simulink model "model"  (R2014a)
(part 5 of 5)

  T_195060971_110000_Подстанция_«Игольская»/RConn1 -- L_195060971/LConn1
  T_195060971_110000_Подстанция_«Игольская»/RConn2 -- L_195060971/LConn2
  L_195060971/LConn3 -- T_195060971_110000_Подстанция_«Игольская»/RConn3 -- bus396/LConn1
  T_332123970__/RConn1 -- L_332123970/LConn1
  T_332123970__/RConn2 -- L_332123970/LConn2
  L_332123970/LConn3 -- T_332123970__/RConn3 -- bus397/LConn1
  T_332122569__/RConn1 -- L_332122569/LConn1
  T_332122569__/RConn2 -- L_332122569/LConn2
  L_332122569/LConn3 -- T_332122569__/RConn3 -- bus398/LConn1
  T_194874204_110000_Подстанция_«Крапивинская»/RConn1 -- L_194874204/LConn1
  T_194874204_110000_Подстанция_«Крапивинская»/RConn2 -- L_194874204/LConn2
  L_194874204/LConn3 -- T_194874204_110000_Подстанция_«Крапивинская»/RConn3 -- bus399/LConn1
  T_100718452__Ефремовская/RConn1 -- L_100718452/LConn1
  T_100718452__Ефремовская/RConn2 -- L_100718452/LConn2
  L_100718452/LConn3 -- T_100718452__Ефремовская/RConn3 -- bus400/LConn1
  T_94337786__Оловозаводская/RConn1 -- L_94337786/LConn1
  T_94337786__Оловозаводская/RConn2 -- L_94337786/LConn2
  L_94337786/LConn3 -- T_94337786__Оловозаводская/RConn3 -- bus401/LConn1
  T_201600394_110000_Подстанция_«Верх_Угрюм»/RConn1 -- L_201600394/LConn1
  T_201600394_110000_Подстанция_«Верх_Угрюм»/RConn2 -- L_201600394/LConn2
  L_201600394/LConn3 -- T_201600394_110000_Подстанция_«Верх_Угрюм»/RConn3 -- bus402/LConn1
  T_203056539__Тяговая_ПС_Суховская/RConn1 -- L_203056539/LConn1
  T_203056539__Тяговая_ПС_Суховская/RConn2 -- L_203056539/LConn2
  L_203056539/LConn3 -- T_203056539__Тяговая_ПС_Суховская/RConn3 -- bus403/LConn1
  T_298817867__/RConn1 -- L_298817867/LConn1
  T_298817867__/RConn2 -- L_298817867/LConn2
  L_298817867/LConn3 -- T_298817867__/RConn3 -- bus404/LConn1
  T_367574444__/RConn1 -- L_367574444/LConn1
  T_367574444__/RConn2 -- L_367574444/LConn2
  L_367574444/LConn3 -- T_367574444__/RConn3 -- bus405/LConn1
  T_283373486__/RConn1 -- L_283373486/LConn1
  T_283373486__/RConn2 -- L_283373486/LConn2
  L_283373486/LConn3 -- T_283373486__/RConn3 -- bus406/LConn1
  "T_110542603_220000_ПС_№152_\"Новокрасноярская\""/RConn1 -- L_110542603/LConn1
  "T_110542603_220000_ПС_№152_\"Новокрасноярская\""/RConn2 -- L_110542603/LConn2
  L_110542603/LConn3 -- "T_110542603_220000_ПС_№152_\"Новокрасноярская\""/RConn3 -- bus407/LConn1
  T_116607512__/RConn1 -- L_116607512/LConn1
  T_116607512__/RConn2 -- L_116607512/LConn2
  L_116607512/LConn3 -- T_116607512__/RConn3 -- bus408/LConn1
  T_394149419_220000_Подстанция_«Орловка»/RConn1 -- L_394149419/LConn1
  T_394149419_220000_Подстанция_«Орловка»/RConn2 -- L_394149419/LConn2
  L_394149419/LConn3 -- T_394149419_220000_Подстанция_«Орловка»/RConn3 -- bus409/LConn1
  T_166018985_500000_Подстанция_«Томская»/RConn1 -- L_166018985/LConn1
  T_166018985_500000_Подстанция_«Томская»/RConn2 -- L_166018985/LConn2
  L_166018985/LConn3 -- T_166018985_500000_Подстанция_«Томская»/RConn3 -- bus410/LConn1
  T_48050742_220000_ПС_ЦРП_220_кВ/RConn1 -- L_48050742/LConn1
  T_48050742_220000_ПС_ЦРП_220_кВ/RConn2 -- L_48050742/LConn2
  L_48050742/LConn3 -- T_48050742_220000_ПС_ЦРП_220_кВ/RConn3 -- bus411/LConn1
  T_220574879_220000_ОРУ___ГПП_3/RConn1 -- L_220574879/LConn1
  T_220574879_220000_ОРУ___ГПП_3/RConn2 -- L_220574879/LConn2
  L_220574879/LConn3 -- T_220574879_220000_ОРУ___ГПП_3/RConn3 -- bus412/LConn1
  T_60040500_220000_ОРУ___ГПП_5/RConn1 -- L_60040500/LConn1
  T_60040500_220000_ОРУ___ГПП_5/RConn2 -- L_60040500/LConn2
  L_60040500/LConn3 -- T_60040500_220000_ОРУ___ГПП_5/RConn3 -- bus413/LConn1
  T_60040415_220000_ОРУ___ГПП_1/RConn1 -- L_60040415/LConn1
  T_60040415_220000_ОРУ___ГПП_1/RConn2 -- L_60040415/LConn2
  L_60040415/LConn3 -- T_60040415_220000_ОРУ___ГПП_1/RConn3 -- bus414/LConn1
  "T_105828925_220000;110000;10000_ПС_\"Узловая\""/RConn1 -- L_105828925/LConn1
  "T_105828925_220000;110000;10000_ПС_\"Узловая\""/RConn2 -- L_105828925/LConn2
  L_105828925/LConn3 -- "T_105828925_220000;110000;10000_ПС_\"Узловая\""/RConn3 -- bus415/LConn1
  T_435735615_220000_ОРУ_220_кВ/RConn1 -- L_435735615/LConn1
  T_435735615_220000_ОРУ_220_кВ/RConn2 -- L_435735615/LConn2
  L_435735615/LConn3 -- T_435735615_220000_ОРУ_220_кВ/RConn3 -- bus416/LConn1
  T_221635306__Подстанция_«Сорская»/RConn1 -- L_221635306/LConn1
  T_221635306__Подстанция_«Сорская»/RConn2 -- L_221635306/LConn2
  L_221635306/LConn3 -- T_221635306__Подстанция_«Сорская»/RConn3 -- bus417/LConn1
  T_228972838__/RConn1 -- L_228972838/LConn1
  T_228972838__/RConn2 -- L_228972838/LConn2
  L_228972838/LConn3 -- T_228972838__/RConn3 -- bus418/LConn1
  T_113629981_220000;110000;35000;fixme_/RConn1 -- L_113629981/LConn1
  T_113629981_220000;110000;35000;fixme_/RConn2 -- L_113629981/LConn2
  L_113629981/LConn3 -- T_113629981_220000;110000;35000;fixme_/RConn3 -- bus419/LConn1
  T_228023756_220000_Подстанция_«Вертикос»/RConn1 -- L_228023756/LConn1
  T_228023756_220000_Подстанция_«Вертикос»/RConn2 -- L_228023756/LConn2
  L_228023756/LConn3 -- T_228023756_220000_Подстанция_«Вертикос»/RConn3 -- bus420/LConn1
  T_245816959__/RConn1 -- L_245816959/LConn1
  T_245816959__/RConn2 -- L_245816959/LConn2
  L_245816959/LConn3 -- T_245816959__/RConn3 -- bus421/LConn1
  T_60040328_220000_ОРУ___ГПП_4/RConn1 -- L_60040328/LConn1
  T_60040328_220000_ОРУ___ГПП_4/RConn2 -- L_60040328/LConn2
  L_60040328/LConn3 -- T_60040328_220000_ОРУ___ГПП_4/RConn3 -- bus422/LConn1
  T_116489400__/RConn1 -- L_116489400/LConn1
  T_116489400__/RConn2 -- L_116489400/LConn2
  L_116489400/LConn3 -- T_116489400__/RConn3 -- bus423/LConn1
  T_60040606_220000_ОРУ___ГПП_2/RConn1 -- L_60040606/LConn1
  T_60040606_220000_ОРУ___ГПП_2/RConn2 -- L_60040606/LConn2
  L_60040606/LConn3 -- T_60040606_220000_ОРУ___ГПП_2/RConn3 -- bus424/LConn1
  T_341189940__/RConn1 -- L_341189940/LConn1
  T_341189940__/RConn2 -- L_341189940/LConn2
  L_341189940/LConn3 -- T_341189940__/RConn3 -- bus425/LConn1
  T_166616387__ЭС_2_СХК/RConn1 -- L_166616387/LConn1
  T_166616387__ЭС_2_СХК/RConn2 -- L_166616387/LConn2
  L_166616387/LConn3 -- T_166616387__ЭС_2_СХК/RConn3 -- bus426/LConn1
  T_131753194_220000;110000;10000_Абакан_Районная/RConn1 -- L_131753194/LConn1
  T_131753194_220000;110000;10000_Абакан_Районная/RConn2 -- L_131753194/LConn2
  L_131753194/LConn3 -- T_131753194_220000;110000;10000_Абакан_Районная/RConn3 -- bus427/LConn1
  T_115163974_220000_Подстанция_«Минусинск_Опорная»/RConn1 -- L_115163974/LConn1
  T_115163974_220000_Подстанция_«Минусинск_Опорная»/RConn2 -- L_115163974/LConn2
  L_115163974/LConn3 -- T_115163974_220000_Подстанция_«Минусинск_Опорная»/RConn3 -- bus428/LConn1
  "T_60040448_220000_РПС_\"КРАМЗ\""/RConn1 -- L_60040448/LConn1
  "T_60040448_220000_РПС_\"КРАМЗ\""/RConn2 -- L_60040448/LConn2
  L_60040448/LConn3 -- "T_60040448_220000_РПС_\"КРАМЗ\""/RConn3 -- bus429/LConn1
  T_308372785_220000_/RConn1 -- L_308372785/LConn1
  T_308372785_220000_/RConn2 -- L_308372785/LConn2
  L_308372785/LConn3 -- T_308372785_220000_/RConn3 -- bus430/LConn1
  T_308372786_220000_/RConn1 -- L_308372786/LConn1
  T_308372786_220000_/RConn2 -- L_308372786/LConn2
  L_308372786/LConn3 -- T_308372786_220000_/RConn3 -- bus431/LConn1
  T_60040627_220000_/RConn1 -- L_60040627/LConn1
  T_60040627_220000_/RConn2 -- L_60040627/LConn2
  L_60040627/LConn3 -- T_60040627_220000_/RConn3 -- bus432/LConn1
  "T_81603854__ПС_220_кВ_\"Урожай\""/RConn1 -- L_81603854/LConn1
  "T_81603854__ПС_220_кВ_\"Урожай\""/RConn2 -- L_81603854/LConn2
  L_81603854/LConn3 -- "T_81603854__ПС_220_кВ_\"Урожай\""/RConn3 -- bus433/LConn1
  T_88364440_220000_Подстанция_«Карасук_3_(тяговая)»/RConn1 -- L_88364440/LConn1
  T_88364440_220000_Подстанция_«Карасук_3_(тяговая)»/RConn2 -- L_88364440/LConn2
  L_88364440/LConn3 -- T_88364440_220000_Подстанция_«Карасук_3_(тяговая)»/RConn3 -- bus434/LConn1
  T_240874260__/RConn1 -- L_240874260/LConn1
  T_240874260__/RConn2 -- L_240874260/LConn2
  L_240874260/LConn3 -- T_240874260__/RConn3 -- bus435/LConn1
  T_290406343__/RConn1 -- L_290406343/LConn1
  T_290406343__/RConn2 -- L_290406343/LConn2
  L_290406343/LConn3 -- T_290406343__/RConn3 -- bus436/LConn1
  T_271058766__/RConn1 -- L_271058766/LConn1
  T_271058766__/RConn2 -- L_271058766/LConn2
  L_271058766/LConn3 -- T_271058766__/RConn3 -- bus437/LConn1
  T_166616386__ЭС_2_СХК/RConn1 -- L_166616386/LConn1
  T_166616386__ЭС_2_СХК/RConn2 -- L_166616386/LConn2
  L_166616386/LConn3 -- T_166616386__ЭС_2_СХК/RConn3 -- bus438/LConn1
  T_228960140__/RConn1 -- L_228960140/LConn1
  T_228960140__/RConn2 -- L_228960140/LConn2
  L_228960140/LConn3 -- T_228960140__/RConn3 -- bus439/LConn1
  T_60040659_220000_ОРУ___ГПП_6/RConn1 -- L_60040659/LConn1
  T_60040659_220000_ОРУ___ГПП_6/RConn2 -- L_60040659/LConn2
  L_60040659/LConn3 -- T_60040659_220000_ОРУ___ГПП_6/RConn3 -- bus440/LConn1
  T_130503101_220000_Подстанция_«Советско_Соснинская»/RConn1 -- L_130503101/LConn1
  T_130503101_220000_Подстанция_«Советско_Соснинская»/RConn2 -- L_130503101/LConn2
  L_130503101/LConn3 -- T_130503101_220000_Подстанция_«Советско_Соснинская»/RConn3 -- bus441/LConn1
  T_223947264_500000_Подстанция_«Алюминиевая»/RConn1 -- L_223947264/LConn1
  T_223947264_500000_Подстанция_«Алюминиевая»/RConn2 -- L_223947264/LConn2
  L_223947264/LConn3 -- T_223947264_500000_Подстанция_«Алюминиевая»/RConn3 -- bus442/LConn1
  T_227781890_500000_КРУЭ_500_кВ/RConn1 -- L_227781890/LConn1
  T_227781890_500000_КРУЭ_500_кВ/RConn2 -- L_227781890/LConn2
  L_227781890/LConn3 -- T_227781890_500000_КРУЭ_500_кВ/RConn3 -- bus443/LConn1
  T_227781922_500000_ОРУ_500_кВ/RConn1 -- L_227781922/LConn1
  T_227781922_500000_ОРУ_500_кВ/RConn2 -- L_227781922/LConn2
  L_227781922/LConn3 -- T_227781922_500000_ОРУ_500_кВ/RConn3 -- bus444/LConn1
  T_225711294_500000;220000_Братский_переключательный_пункт/RConn1 -- L_225711294/LConn1
  T_225711294_500000;220000_Братский_переключательный_пункт/RConn2 -- L_225711294/LConn2
  L_225711294/LConn3 -- T_225711294_500000;220000_Братский_переключательный_пункт/RConn3 -- bus445/LConn1
  T_157280374_500000_ПС_Новокузнецкая_500_кВ/RConn1 -- L_157280374/LConn1
  T_157280374_500000_ПС_Новокузнецкая_500_кВ/RConn2 -- L_157280374/LConn2
  L_157280374/LConn3 -- T_157280374_500000_ПС_Новокузнецкая_500_кВ/RConn3 -- bus446/LConn1
  T_131767848_500000;110000;35000_Тайшет/RConn1 -- L_131767848/LConn1
  T_131767848_500000;110000;35000_Тайшет/RConn2 -- L_131767848/LConn2
  L_131767848/LConn3 -- T_131767848_500000;110000;35000_Тайшет/RConn3 -- bus447/LConn1
  T_97377449_500000_Подстанция_«Барабинская»/RConn1 -- L_97377449/LConn1
  T_97377449_500000_Подстанция_«Барабинская»/RConn2 -- L_97377449/LConn2
  L_97377449/LConn3 -- T_97377449_500000_Подстанция_«Барабинская»/RConn3 -- bus448/LConn1
  T_107673466_500000;220000_Подстанция_«Таврическая»/RConn1 -- L_107673466/LConn1
  T_107673466_500000;220000_Подстанция_«Таврическая»/RConn2 -- L_107673466/LConn2
  L_107673466/LConn3 -- T_107673466_500000;220000_Подстанция_«Таврическая»/RConn3 -- bus449/LConn1
  T_100584107_500000_Подстанция_«Алтай»/RConn1 -- L_100584107/LConn1
  T_100584107_500000_Подстанция_«Алтай»/RConn2 -- L_100584107/LConn2
  L_100584107/LConn3 -- T_100584107_500000_Подстанция_«Алтай»/RConn3 -- bus450/LConn1
  T_100584147_500000_Подстанция_«Барнаульская»/RConn1 -- L_100584147/LConn1
  T_100584147_500000_Подстанция_«Барнаульская»/RConn2 -- L_100584147/LConn2
  L_100584147/LConn3 -- T_100584147_500000_Подстанция_«Барнаульская»/RConn3 -- bus451/LConn1
  "T_122224559_500000;220000;110000_ПС_500_кВ_\"Иртышская\""/RConn1 -- L_122224559/LConn1
  "T_122224559_500000;220000;110000_ПС_500_кВ_\"Иртышская\""/RConn2 -- L_122224559/LConn2
  L_122224559/LConn3 -- "T_122224559_500000;220000;110000_ПС_500_кВ_\"Иртышская\""/RConn3 -- bus452/LConn1
  T_228246728_500000;220000_/RConn1 -- L_228246728/LConn1
  T_228246728_500000;220000_/RConn2 -- L_228246728/LConn2
  L_228246728/LConn3 -- T_228246728_500000;220000_/RConn3 -- bus453/LConn1
